simulink model "lesssimple"  (Simulink 7.2)
settings: Solver=FixedStepDiscrete  StartTime=0.0  StopTime=inf  FixedStep=0.1  RelTol=1e-3
libraries: SimvtkRenderingLibrary x8, SimvtkGraphicsLibrary x3, SimvtkIOLibrary x1
settings Model: Creator=acampi  LastModifiedBy=dgobbi
settings OptimizationCC: InitFltsAndDblsToZero=on
settings DebuggingCC: SaveWithParameterizedLinksMsg=none

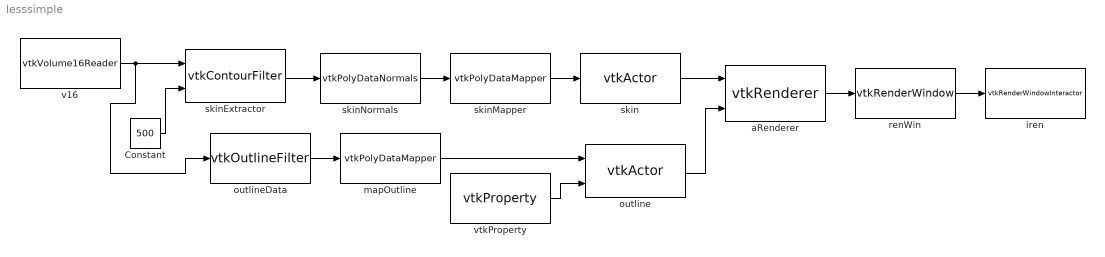
== system lesssimple ==
  Constant : Constant  Value=500  OutDataType=sfix(16)  OutScaling=2^0
  aRenderer : SimvtkRenderingLibrary/vtkRenderer  VTKInputSelf=off  VTKInputActiveCamera=off  VTKInputActor=2  VTKInputActor2D=0  VTKInputCuller=0  VTKInputDelegate=off  VTKInputLight=0  VTKInputProp=0  VTKInputViewProp=0  VTKInputVolume=0  AllocatedRenderTimeInputIndicator=Use Default  VTKParamAllocatedRenderTime=0  AmbientInputIndicator=Use Default  VTKParamAmbient=[0,0,0]  AspectInputIndicator=Use Default  VTKParamAspect=[0,0]  AutomaticLightCreationInputIndicator=Use Default  VTKParamAutomaticLightCreation=0  BackgroundInputIndicator=As Parameter  VTKParamBackground=[0.5,0.5,1]  Background2InputIndicator=Use Default  VTKParamBackground2=[0,0,0]  BackingStoreInputIndicator=Use Default  VTKParamBackingStore=0  DisplayPointInputIndicator=Use Default  VTKParamDisplayPoint=[0,0,0]  DrawInputIndicator=Use Default  VTKParamDraw=0  EraseInputIndicator=Use Default  VTKParamErase=0  GradientBackgroundInputIndicator=Use Default  VTKParamGradientBackground=0  InteractiveInputIndicator=Use Default  VTKParamInteractive=0  IsPickingInputIndicator=off  VTKParamIsPicking=0  LastRenderTimeInSecondsInputIndicator=off  VTKParamLastRenderTimeInSeconds=0  LastRenderingUsedDepthPeelingInputIndicator=off  VTKParamLastRenderingUsedDepthPeeling=0  LayerInputIndicator=Use Default  VTKParamLayer=0  LightFollowCameraInputIndicator=Use Default  VTKParamLightFollowCamera=0  MaximumNumberOfPeelsInputIndicator=Use Default  VTKParamMaximumNumberOfPeels=0  NearClippingPlaneToleranceInputIndicator=Use Default  VTKParamNearClippingPlaneTolerance=0  NearClippingPlaneToleranceMaxValueInputIndicator=off  VTKParamNearClippingPlaneToleranceMaxValue=0  NearClippingPlaneToleranceMinValueInputIndicator=off  VTKParamNearClippingPlaneToleranceMinValue=0  NumberOfPropsRenderedInputIndicator=off  VTKParamNumberOfPropsRendered=0  OcclusionRatioInputIndicator=Use Default  VTKParamOcclusionRatio=0  OcclusionRatioMaxValueInputIndicator=off  VTKParamOcclusionRatioMaxValue=0  OcclusionRatioMinValueInputIndicator=off  VTKParamOcclusionRatioMinValue=0  PickHeightInputIndicator=off  VTKParamPickHeight=0  PickWidthInputIndicator=off  VTKParamPickWidth=0  PickXInputIndicator=off  VTKParamPickX=0  PickX1InputIndicator=off  VTKParamPickX1=0  PickX2InputIndicator=off  VTKParamPickX2=0  PickYInputIndicator=off  VTKParamPickY=0  PickY1InputIndicator=off  VTKParamPickY1=0  PickY2InputIndicator=off  VTKParamPickY2=0  PickedZInputIndicator=off  VTKParamPickedZ=0  PixelAspectInputIndicator=Use Default  VTKParamPixelAspect=[0,0]  PreserveDepthBufferInputIndicator=Use Default  VTKParamPreserveDepthBuffer=0  TiledAspectRatioInputIndicator=off  VTKParamTiledAspectRatio=0  TimeFactorInputIndicator=off  VTKParamTimeFactor=0  TwoSidedLightingInputIndicator=Use Default  VTKParamTwoSidedLighting=0  UseDepthPeelingInputIndicator=Use Default  VTKParamUseDepthPeeling=0  ViewPointInputIndicator=Use Default  VTKParamViewPoint=[0,0,0]  ViewportInputIndicator=Use Default  VTKParamViewport=[0,0,0,0]  WorldPointInputIndicator=Use Default  VTKParamWorldPoint=[0,0,0,0]  VTKOutputSelf=on  VTKOutputActors=off  VTKOutputActors2D=off  VTKOutputCullers=off  VTKOutputLights=off  VTKOutputPickResultProps=off  VTKOutputProps=off  VTKOutputSelector=off  VTKOutputVTKWindow=off  VTKOutputViewProps=off  VTKOutputVolumes=off
  iren : SimvtkRenderingLibrary/vtkRenderWindowInteractor  VTKInputSelf=off  VTKInputInteractorStyle=off  VTKInputPicker=off  VTKInputRenderWindow=on  AltKeyInputIndicator=Use Default  VTKParamAltKey=0  ControlKeyInputIndicator=Use Default  VTKParamControlKey=0  DesiredUpdateRateInputIndicator=Use Default  VTKParamDesiredUpdateRate=0  DesiredUpdateRateMaxValueInputIndicator=off  VTKParamDesiredUpdateRateMaxValue=0  DesiredUpdateRateMinValueInputIndicator=off  VTKParamDesiredUpdateRateMinValue=0  DollyInputIndicator=Use Default  VTKParamDolly=0  EnableRenderInputIndicator=Use Default  VTKParamEnableRender=0  EnabledInputIndicator=off  VTKParamEnabled=0  EventPositionInputIndicator=Use Default  VTKParamEventPosition=[0,0]  EventPositionFlipYInputIndicator=Use Default  VTKParamEventPositionFlipY=[0,0]  EventSizeInputIndicator=Use Default  VTKParamEventSize=[0,0]  InitializedInputIndicator=off  VTKParamInitialized=0  KeyCodeInputIndicator=Use Default  VTKParamKeyCode=0  KeySymInputIndicator=Use Default  VTKParamKeySym=0  LastEventPositionInputIndicator=Use Default  VTKParamLastEventPosition=[0,0]  LightFollowCameraInputIndicator=Use Default  VTKParamLightFollowCamera=0  NumberOfFlyFramesInputIndicator=Use Default  VTKParamNumberOfFlyFrames=0  NumberOfFlyFramesMaxValueInputIndicator=off  VTKParamNumberOfFlyFramesMaxValue=0  NumberOfFlyFramesMinValueInputIndicator=off  VTKParamNumberOfFlyFramesMinValue=0  RepeatCountInputIndicator=Use Default  VTKParamRepeatCount=0  ShiftKeyInputIndicator=Use Default  VTKParamShiftKey=0  SizeInputIndicator=Use Default  VTKParamSize=[0,0]  StillUpdateRateInputIndicator=Use Default  VTKParamStillUpdateRate=0  StillUpdateRateMaxValueInputIndicator=off  VTKParamStillUpdateRateMaxValue=0  StillUpdateRateMinValueInputIndicator=off  VTKParamStillUpdateRateMinValue=0  TimerDurationInputIndicator=Use Default  VTKParamTimerDuration=0  TimerDurationMaxValueInputIndicator=off  VTKParamTimerDurationMaxValue=0  TimerDurationMinValueInputIndicator=off  VTKParamTimerDurationMinValue=0  TimerEventDurationInputIndicator=Use Default  VTKParamTimerEventDuration=0  TimerEventIdInputIndicator=Use Default  VTKParamTimerEventId=0  TimerEventPlatformIdInputIndicator=Use Default  VTKParamTimerEventPlatformId=0  TimerEventTypeInputIndicator=Use Default  VTKParamTimerEventType=0  VTKOutputSelf=off  VTKOutputObserverMediator=off
  mapOutline : SimvtkRenderingLibrary/vtkPolyDataMapper  VTKInputSelf=off  VTKInputClippingPlane=0  VTKInputClippingPlanes=off  VTKInputLookupTable=off  ArrayAccessModeInputIndicator=off  VTKParamArrayAccessMode=0  ArrayComponentInputIndicator=off  VTKParamArrayComponent=0  ArrayIdInputIndicator=off  VTKParamArrayId=0  ArrayNameInputIndicator=off  VTKParamArrayName=0  ColorModeInputIndicator=Use Default  VTKParamColorMode=0  ColorModeAsStringInputIndicator=off  VTKParamColorModeAsString=0  GhostLevelInputIndicator=Use Default  VTKParamGhostLevel=0  ImmediateModeRenderingInputIndicator=Use Default  VTKParamImmediateModeRendering=0  InterpolateScalarsBeforeMappingInputIndicator=Use Default  VTKParamInterpolateScalarsBeforeMapping=0  LengthInputIndicator=off  VTKParamLength=0  NumberOfPiecesInputIndicator=Use Default  VTKParamNumberOfPieces=0  NumberOfSubPiecesInputIndicator=Use Default  VTKParamNumberOfSubPieces=0  PieceInputIndicator=Use Default  VTKParamPiece=0  RenderTimeInputIndicator=Use Default  VTKParamRenderTime=0  ScalarMaterialModeInputIndicator=Use Default  VTKParamScalarMaterialMode=0  ScalarMaterialModeAsStringInputIndicator=off  VTKParamScalarMaterialModeAsString=0  ScalarModeInputIndicator=Use Default  VTKParamScalarMode=0  ScalarModeAsStringInputIndicator=off  VTKParamScalarModeAsString=0  ScalarRangeInputIndicator=Use Default  VTKParamScalarRange=[0,0]  ScalarVisibilityInputIndicator=Use Default  VTKParamScalarVisibility=0  StaticInputIndicator=Use Default  VTKParamStatic=0  SupportsSelectionInputIndicator=off  VTKParamSupportsSelection=0  TimeToDrawInputIndicator=off  VTKParamTimeToDraw=0  UseLookupTableScalarRangeInputIndicator=Use Default  VTKParamUseLookupTableScalarRange=0  VTKOutputSelf=on
  outline : SimvtkRenderingLibrary/vtkActor  VTKInputSelf=off  VTKInputBackfaceProperty=off  VTKInputMapper=on  VTKInputProperty=on  VTKInputPropertyKeys=off  VTKInputTexture=off  VTKInputUserMatrix=off  VTKInputUserTransform=off  DragableInputIndicator=Use Default  VTKParamDragable=0  IsIdentityInputIndicator=off  VTKParamIsIdentity=0  LengthInputIndicator=off  VTKParamLength=0  NumberOfPartsInputIndicator=off  VTKParamNumberOfParts=0  NumberOfPathsInputIndicator=off  VTKParamNumberOfPaths=0  OrientationInputIndicator=Use Default  VTKParamOrientation=[0,0,0]  OriginInputIndicator=Use Default  VTKParamOrigin=[0,0,0]  PickableInputIndicator=Use Default  VTKParamPickable=0  PositionInputIndicator=Use Default  VTKParamPosition=[0,0,0]  RedrawMTimeInputIndicator=off  VTKParamRedrawMTime=0  ScaleInputIndicator=Use Default  VTKParamScale=[0,0,0]  SupportsSelectionInputIndicator=off  VTKParamSupportsSelection=0  UseBoundsInputIndicator=Use Default  VTKParamUseBounds=0  UserTransformMatrixMTimeInputIndicator=off  VTKParamUserTransformMatrixMTime=0  VisibilityInputIndicator=Use Default  VTKParamVisibility=0  VTKOutputSelf=on  VTKOutputMatrix=off  VTKOutputNextPart=off  VTKOutputNextPath=off
  outlineData : SimvtkGraphicsLibrary/vtkOutlineFilter  VTKInputSelf=off  VTKOutputSelf=off
  renWin : SimvtkRenderingLibrary/vtkRenderWindow  VTKInputSelf=off  VTKInputInteractor=off  VTKInputRenderer=1  AAFramesInputIndicator=Use Default  VTKParamAAFrames=0  AbortRenderInputIndicator=Use Default  VTKParamAbortRender=0  AlphaBitPlanesInputIndicator=Use Default  VTKParamAlphaBitPlanes=0  AnaglyphColorMaskInputIndicator=Use Default  VTKParamAnaglyphColorMask=[0,0]  AnaglyphColorSaturationInputIndicator=Use Default  VTKParamAnaglyphColorSaturation=0  AnaglyphColorSaturationMaxValueInputIndicator=off  VTKParamAnaglyphColorSaturationMaxValue=0  AnaglyphColorSaturationMinValueInputIndicator=off  VTKParamAnaglyphColorSaturationMinValue=0  BordersInputIndicator=Use Default  VTKParamBorders=0  CurrentCursorInputIndicator=Use Default  VTKParamCurrentCursor=0  CursorPositionInputIndicator=Use Default  VTKParamCursorPosition=[0,0]  DPIInputIndicator=Use Default  VTKParamDPI=0  DPIMaxValueInputIndicator=off  VTKParamDPIMaxValue=0  DPIMinValueInputIndicator=off  VTKParamDPIMinValue=0  DepthBufferSizeInputIndicator=off  VTKParamDepthBufferSize=0  DesiredUpdateRateInputIndicator=Use Default  VTKParamDesiredUpdateRate=0  DoubleBufferInputIndicator=Use Default  VTKParamDoubleBuffer=0  EraseInputIndicator=Use Default  VTKParamErase=0  EventPendingInputIndicator=off  VTKParamEventPending=0  FDFramesInputIndicator=Use Default  VTKParamFDFrames=0  FullScreenInputIndicator=Use Default  VTKParamFullScreen=0  InAbortCheckInputIndicator=Use Default  VTKParamInAbortCheck=0  IsPickingInputIndicator=Use Default  VTKParamIsPicking=0  LastGraphicErrorStringInputIndicator=off  VTKParamLastGraphicErrorString=0  LineSmoothingInputIndicator=Use Default  VTKParamLineSmoothing=0  MappedInputIndicator=Use Default  VTKParamMapped=0  MultiSamplesInputIndicator=Use Default  VTKParamMultiSamples=0  NeverRenderedInputIndicator=off  VTKParamNeverRendered=0  NextWindowInfoInputIndicator=Use Default  VTKParamNextWindowInfo=0  NumberOfLayersInputIndicator=Use Default  VTKParamNumberOfLayers=0  NumberOfLayersMaxValueInputIndicator=off  VTKParamNumberOfLayersMaxValue=0  NumberOfLayersMinValueInputIndicator=off  VTKParamNumberOfLayersMinValue=0  OffScreenRenderingInputIndicator=Use Default  VTKParamOffScreenRendering=0  ParentInfoInputIndicator=Use Default  VTKParamParentInfo=0  PointSmoothingInputIndicator=Use Default  VTKParamPointSmoothing=0  PolygonSmoothingInputIndicator=Use Default  VTKParamPolygonSmoothing=0  PositionInputIndicator=Use Default  VTKParamPosition=[0,0]  RenderLibraryInputIndicator=off  VTKParamRenderLibrary=0  ReportGraphicErrorsInputIndicator=Use Default  VTKParamReportGraphicErrors=0  SizeInputIndicator=Use Default  VTKParamSize=[640,640]  StencilCapableInputIndicator=Use Default  VTKParamStencilCapable=0  StereoCapableWindowInputIndicator=Use Default  VTKParamStereoCapableWindow=0  StereoRenderInputIndicator=Use Default  VTKParamStereoRender=0  StereoTypeInputIndicator=Use Default  VTKParamStereoType=0  StereoTypeAsStringInputIndicator=off  VTKParamStereoTypeAsString=0  SubFramesInputIndicator=Use Default  VTKParamSubFrames=0  SwapBuffersInputIndicator=Use Default  VTKParamSwapBuffers=0  TileScaleInputIndicator=Use Default  VTKParamTileScale=[0,0]  TileViewportInputIndicator=Use Default  VTKParamTileViewport=[0,0,0,0]  WindowInfoInputIndicator=Use Default  VTKParamWindowInfo=0  WindowNameInputIndicator=Use Default  VTKParamWindowName=0  VTKOutputSelf=on  VTKOutputPainterDeviceAdapter=off  VTKOutputRenderers=off
  skin : SimvtkRenderingLibrary/vtkActor  VTKInputSelf=off  VTKInputBackfaceProperty=off  VTKInputMapper=on  VTKInputProperty=off  VTKInputPropertyKeys=off  VTKInputTexture=off  VTKInputUserMatrix=off  VTKInputUserTransform=off  DragableInputIndicator=Use Default  VTKParamDragable=0  IsIdentityInputIndicator=off  VTKParamIsIdentity=0  LengthInputIndicator=off  VTKParamLength=0  NumberOfPartsInputIndicator=off  VTKParamNumberOfParts=0  NumberOfPathsInputIndicator=off  VTKParamNumberOfPaths=0  OrientationInputIndicator=Use Default  VTKParamOrientation=[0,0,0]  OriginInputIndicator=Use Default  VTKParamOrigin=[0,0,0]  PickableInputIndicator=Use Default  VTKParamPickable=0  PositionInputIndicator=Use Default  VTKParamPosition=[0,0,0]  RedrawMTimeInputIndicator=off  VTKParamRedrawMTime=0  ScaleInputIndicator=Use Default  VTKParamScale=[0,0,0]  SupportsSelectionInputIndicator=off  VTKParamSupportsSelection=0  UseBoundsInputIndicator=Use Default  VTKParamUseBounds=0  UserTransformMatrixMTimeInputIndicator=off  VTKParamUserTransformMatrixMTime=0  VisibilityInputIndicator=Use Default  VTKParamVisibility=0  VTKOutputSelf=on  VTKOutputMatrix=off  VTKOutputNextPart=off  VTKOutputNextPath=off
  skinExtractor : SimvtkGraphicsLibrary/vtkContourFilter  VTKInputSelf=off  VTKInputLocator=off  VTKInputScalarTree=off  ArrayComponentInputIndicator=Use Default  VTKParamArrayComponent=0  ComputeGradientsInputIndicator=Use Default  VTKParamComputeGradients=0  ComputeNormalsInputIndicator=Use Default  VTKParamComputeNormals=0  ComputeScalarsInputIndicator=Use Default  VTKParamComputeScalars=0  NumberOfContoursInputIndicator=Use Default  VTKParamNumberOfContours=0  UseScalarTreeInputIndicator=Use Default  VTKParamUseScalarTree=0  ValueInputIndicator=As Input  VTKParamValue=1  VTKOutputSelf=off
  skinMapper : SimvtkRenderingLibrary/vtkPolyDataMapper  VTKInputSelf=off  VTKInputClippingPlane=0  VTKInputClippingPlanes=off  VTKInputLookupTable=off  ArrayAccessModeInputIndicator=off  VTKParamArrayAccessMode=0  ArrayComponentInputIndicator=off  VTKParamArrayComponent=0  ArrayIdInputIndicator=off  VTKParamArrayId=0  ArrayNameInputIndicator=off  VTKParamArrayName=0  ColorModeInputIndicator=Use Default  VTKParamColorMode=0  ColorModeAsStringInputIndicator=off  VTKParamColorModeAsString=0  GhostLevelInputIndicator=Use Default  VTKParamGhostLevel=0  ImmediateModeRenderingInputIndicator=Use Default  VTKParamImmediateModeRendering=0  InterpolateScalarsBeforeMappingInputIndicator=Use Default  VTKParamInterpolateScalarsBeforeMapping=0  LengthInputIndicator=off  VTKParamLength=0  NumberOfPiecesInputIndicator=Use Default  VTKParamNumberOfPieces=0  NumberOfSubPiecesInputIndicator=Use Default  VTKParamNumberOfSubPieces=0  PieceInputIndicator=Use Default  VTKParamPiece=0  RenderTimeInputIndicator=Use Default  VTKParamRenderTime=0  ScalarMaterialModeInputIndicator=Use Default  VTKParamScalarMaterialMode=0  ScalarMaterialModeAsStringInputIndicator=off  VTKParamScalarMaterialModeAsString=0  ScalarModeInputIndicator=Use Default  VTKParamScalarMode=0  ScalarModeAsStringInputIndicator=off  VTKParamScalarModeAsString=0  ScalarRangeInputIndicator=Use Default  VTKParamScalarRange=[0,0]  ScalarVisibilityInputIndicator=As Parameter  VTKParamScalarVisibility=0  StaticInputIndicator=Use Default  VTKParamStatic=0  SupportsSelectionInputIndicator=off  VTKParamSupportsSelection=0  TimeToDrawInputIndicator=off  VTKParamTimeToDraw=0  UseLookupTableScalarRangeInputIndicator=Use Default  VTKParamUseLookupTableScalarRange=0  VTKOutputSelf=on
  skinNormals : SimvtkGraphicsLibrary/vtkPolyDataNormals  VTKInputSelf=off  AutoOrientNormalsInputIndicator=Use Default  VTKParamAutoOrientNormals=0  ComputeCellNormalsInputIndicator=Use Default  VTKParamComputeCellNormals=0  ComputePointNormalsInputIndicator=Use Default  VTKParamComputePointNormals=0  ConsistencyInputIndicator=Use Default  VTKParamConsistency=0  FeatureAngleInputIndicator=As Parameter  VTKParamFeatureAngle=60  FeatureAngleMaxValueInputIndicator=off  VTKParamFeatureAngleMaxValue=0  FeatureAngleMinValueInputIndicator=off  VTKParamFeatureAngleMinValue=0  FlipNormalsInputIndicator=Use Default  VTKParamFlipNormals=0  NonManifoldTraversalInputIndicator=Use Default  VTKParamNonManifoldTraversal=0  SplittingInputIndicator=Use Default  VTKParamSplitting=0  VTKOutputSelf=off
  v16 : SimvtkIOLibrary/vtkVolume16Reader  VTKInputSelf=off  VTKInputTransform=off  DataByteOrderInputIndicator=As Parameter  VTKParamDataByteOrder=1  DataByteOrderAsStringInputIndicator=off  VTKParamDataByteOrderAsString=0  DataDimensionsInputIndicator=As Parameter  VTKParamDataDimensions=[64,64]  DataMaskInputIndicator=Use Default  VTKParamDataMask=0  DataOriginInputIndicator=Use Default  VTKParamDataOrigin=[0,0,0]  DataSpacingInputIndicator=As Parameter  VTKParamDataSpacing=[3.2,3.2,1.5]  FilePatternInputIndicator=Use Default  VTKParamFilePattern=0  FilePrefixInputIndicator=As Parameter  VTKParamFilePrefix='Data/headsq/quarter'  HeaderSizeInputIndicator=Use Default  VTKParamHeaderSize=0  ImageRangeInputIndicator=As Parameter  VTKParamImageRange=[1,93]  SwapBytesInputIndicator=Use Default  VTKParamSwapBytes=0  VTKOutputSelf=off
  vtkProperty : SimvtkRenderingLibrary/vtkProperty  VTKInputSelf=off  AmbientInputIndicator=Use Default  VTKParamAmbient=0  AmbientColorInputIndicator=Use Default  VTKParamAmbientColor=[0,0,0]  AmbientMaxValueInputIndicator=off  VTKParamAmbientMaxValue=0  AmbientMinValueInputIndicator=off  VTKParamAmbientMinValue=0  BackfaceCullingInputIndicator=Use Default  VTKParamBackfaceCulling=0  ColorInputIndicator=As Parameter  VTKParamColor=[0,0,0]  DiffuseInputIndicator=Use Default  VTKParamDiffuse=0  DiffuseColorInputIndicator=Use Default  VTKParamDiffuseColor=[0,0,0]  DiffuseMaxValueInputIndicator=off  VTKParamDiffuseMaxValue=0  DiffuseMinValueInputIndicator=off  VTKParamDiffuseMinValue=0  EdgeColorInputIndicator=Use Default  VTKParamEdgeColor=[0,0,0]  EdgeVisibilityInputIndicator=Use Default  VTKParamEdgeVisibility=0  FrontfaceCullingInputIndicator=Use Default  VTKParamFrontfaceCulling=0  InterpolationInputIndicator=Use Default  VTKParamInterpolation=0  InterpolationAsStringInputIndicator=off  VTKParamInterpolationAsString=0  InterpolationMaxValueInputIndicator=off  VTKParamInterpolationMaxValue=0  InterpolationMinValueInputIndicator=off  VTKParamInterpolationMinValue=0  LightingInputIndicator=Use Default  VTKParamLighting=0  LineStipplePatternInputIndicator=Use Default  VTKParamLineStipplePattern=0  LineStippleRepeatFactorInputIndicator=Use Default  VTKParamLineStippleRepeatFactor=0  LineStippleRepeatFactorMaxValueInputIndicator=off  VTKParamLineStippleRepeatFactorMaxValue=0  LineStippleRepeatFactorMinValueInputIndicator=off  VTKParamLineStippleRepeatFactorMinValue=0  LineWidthInputIndicator=Use Default  VTKParamLineWidth=0  LineWidthMaxValueInputIndicator=off  VTKParamLineWidthMaxValue=0  LineWidthMinValueInputIndicator=off  VTKParamLineWidthMinValue=0  NumberOfTexturesInputIndicator=off  VTKParamNumberOfTextures=0  OpacityInputIndicator=Use Default  VTKParamOpacity=0  OpacityMaxValueInputIndicator=off  VTKParamOpacityMaxValue=0  OpacityMinValueInputIndicator=off  VTKParamOpacityMinValue=0  PointSizeInputIndicator=Use Default  VTKParamPointSize=0  PointSizeMaxValueInputIndicator=off  VTKParamPointSizeMaxValue=0  PointSizeMinValueInputIndicator=off  VTKParamPointSizeMinValue=0  RepresentationInputIndicator=Use Default  VTKParamRepresentation=0  RepresentationAsStringInputIndicator=off  VTKParamRepresentationAsString=0  RepresentationMaxValueInputIndicator=off  VTKParamRepresentationMaxValue=0  RepresentationMinValueInputIndicator=off  VTKParamRepresentationMinValue=0  ShadingInputIndicator=Use Default  VTKParamShading=0  SpecularInputIndicator=Use Default  VTKParamSpecular=0  SpecularColorInputIndicator=Use Default  VTKParamSpecularColor=[0,0,0]  SpecularMaxValueInputIndicator=off  VTKParamSpecularMaxValue=0  SpecularMinValueInputIndicator=off  VTKParamSpecularMinValue=0  SpecularPowerInputIndicator=Use Default  VTKParamSpecularPower=0  SpecularPowerMaxValueInputIndicator=off  VTKParamSpecularPowerMaxValue=0  SpecularPowerMinValueInputIndicator=off  VTKParamSpecularPowerMinValue=0  VTKOutputSelf=on  VTKOutputMaterial=off
  wires:
  Constant/1 -> skinExtractor/2
  skinExtractor/1 -> skinNormals/1
  skinNormals/1 -> skinMapper/1
  skinMapper/1 -> skin/1
  outlineData/1 -> mapOutline/1
  mapOutline/1 -> outline/1
  outline/1 -> aRenderer/2
  skin/1 -> aRenderer/1
  aRenderer/1 -> renWin/1
  renWin/1 -> iren/1
  vtkProperty/1 -> outline/2
  v16/1 -> skinExtractor/1, outlineData/1
